simulink model "ModeloUnaOruga"  (R2023b)
settings: Solver=VariableStepAuto  StartTime=0.0  StopTime=10  RelTol=1e-3
model workspace: external: MATLAB File C:\Users\marco\MATLAB\Projects\SimulacionOrugas\Ensamblaje_Sim_v8_DataFile.m (data not in the file)
undefined symbols (not defined in the file or in its folder): smiData, X, Y, Z
libraries: sm_lib x1001, nesl_utility x3, simulink x1
(part 5 of 16)

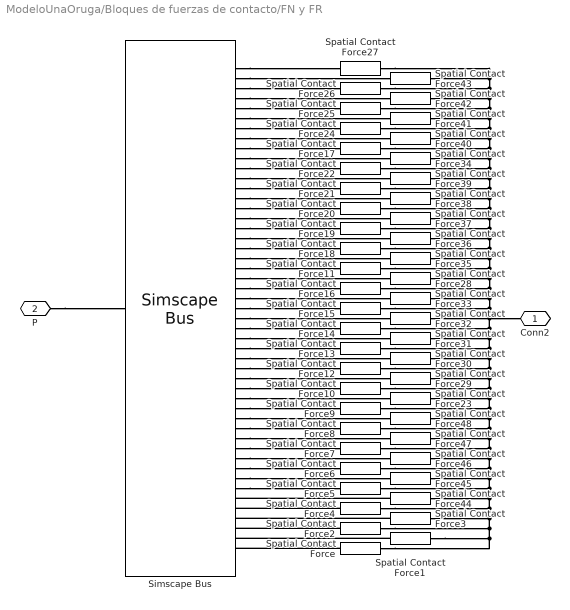
== system ModeloUnaOruga/Bloques de fuerzas de contacto/FN y FR ==
  Simscape Bus : SimscapeBus  HierarchyStrings=Connection49;Connection48;Connection47;Connection46;Connection45;Connection44;Connection43;Connection42;Connection41;Connection40;Connection39;Connection38;Connection37;Connection36;Connection35;Connection34;Connection33;Connection32;Connection31;Connection30;Connection29;Connection28;Connection27;Connection26;Connection25;Connection24;Connection23;Connection22;Connection21;Connection20;Connection19;Connection18;Connection17;Connection16;Connection15;Connection14;Connection13;Connection12;Connection11;Connection10;Connection9;Connection8;Connection7;Connection6;Connection5;Connection4;Connection3;Connection2;Connection1
  Spatial Contact Force{,1..48} (49 alike) : sm_lib/Forces and Torques/Spatial Contact Force  SenseContactBaseRotation=off  SenseContactBaseTranslation=off  CoefficientOfDynamicFriction=0.3  CoefficientOfStaticFriction=0.5  NormalDamping=1e3  NormalDampingUnits=N/(m/s)  SenseContactSignal=off  NormalStiffness=1e6  NormalStiffnessUnits=N/m  FrictionalCriticalVelocity=1e-3  FrictionalCriticalVelocityUnits=m/s  ZeroCrossDetectContactStartAndEnd=off  SenseContactFollowerRotation=off  SenseContactFollowerTranslation=off  FrictionType=SmoothStickSlip  SenseFrictionalForceMagnitude=off  SenseNormalForceMagnitude=off  NormalForceType=SmoothSpringDamper  SenseNormalVelocity=off  SensePenetrationDepth=off  SenseSeparationDistance=off  SenseTangentialVelocity=off  NormalTransitionRegionWidth=1e-4  NormalTransitionRegionWidthUnits=m
  Conn2 : PMIOPort  Side=Right
  P : PMIOPort  Port=2  Side=Left
  connections:
  Spatial Contact Force/RConn1 -- Spatial Contact Force1/RConn1 -- Spatial Contact Force2/RConn1 -- Spatial Contact Force3/RConn1 -- Spatial Contact Force4/RConn1 -- Spatial Contact Force44/RConn1 -- Spatial Contact Force5/RConn1 -- Spatial Contact Force45/RConn1 -- Spatial Contact Force6/RConn1 -- Spatial Contact Force46/RConn1 -- Spatial Contact Force7/RConn1 -- Spatial Contact Force47/RConn1 -- Spatial Contact Force8/RConn1 -- Spatial Contact Force48/RConn1 -- Spatial Contact Force9/RConn1 -- Spatial Contact Force23/RConn1 -- Spatial Contact Force10/RConn1 -- Spatial Contact Force29/RConn1 -- Spatial Contact Force12/RConn1 -- Spatial Contact Force30/RConn1 -- Spatial Contact Force13/RConn1 -- Spatial Contact Force31/RConn1 -- Spatial Contact Force14/RConn1 -- Spatial Contact Force18/RConn1 -- Spatial Contact Force43/RConn1 -- Spatial Contact Force27/RConn1 -- Spatial Contact Force26/RConn1 -- Spatial Contact Force42/RConn1 -- Spatial Contact Force25/RConn1 -- Spatial Contact Force41/RConn1 -- Spatial Contact Force24/RConn1 -- Spatial Contact Force40/RConn1 -- Spatial Contact Force17/RConn1 -- Spatial Contact Force34/RConn1 -- Spatial Contact Force22/RConn1 -- Spatial Contact Force39/RConn1 -- Spatial Contact Force21/RConn1 -- Spatial Contact Force38/RConn1 -- Spatial Contact Force20/RConn1 -- Spatial Contact Force37/RConn1 -- Spatial Contact Force19/RConn1 -- Spatial Contact Force36/RConn1 -- Spatial Contact Force35/RConn1 -- Spatial Contact Force11/RConn1 -- Spatial Contact Force28/RConn1 -- Spatial Contact Force16/RConn1 -- Spatial Contact Force33/RConn1 -- Spatial Contact Force15/RConn1 -- Spatial Contact Force32/RConn1 -- Conn2/RConn1
  Spatial Contact Force/LConn1 -- Simscape Bus/LConn49
  Spatial Contact Force1/LConn1 -- Simscape Bus/LConn48
  Spatial Contact Force2/LConn1 -- Simscape Bus/LConn47
  Spatial Contact Force3/LConn1 -- Simscape Bus/LConn46
  Spatial Contact Force4/LConn1 -- Simscape Bus/LConn45
  Spatial Contact Force44/LConn1 -- Simscape Bus/LConn44
  Simscape Bus/LConn43 -- Spatial Contact Force5/LConn1
  Simscape Bus/LConn42 -- Spatial Contact Force45/LConn1
  Simscape Bus/LConn41 -- Spatial Contact Force6/LConn1
  Simscape Bus/LConn40 -- Spatial Contact Force46/LConn1
  Simscape Bus/LConn39 -- Spatial Contact Force7/LConn1
  Simscape Bus/LConn38 -- Spatial Contact Force47/LConn1
  Simscape Bus/LConn37 -- Spatial Contact Force8/LConn1
  Simscape Bus/LConn36 -- Spatial Contact Force48/LConn1
  Simscape Bus/LConn35 -- Spatial Contact Force9/LConn1
  Simscape Bus/LConn34 -- Spatial Contact Force23/LConn1
  Simscape Bus/LConn33 -- Spatial Contact Force10/LConn1
  Simscape Bus/LConn32 -- Spatial Contact Force29/LConn1
  Simscape Bus/LConn31 -- Spatial Contact Force12/LConn1
  Simscape Bus/LConn30 -- Spatial Contact Force30/LConn1
  Simscape Bus/LConn29 -- Spatial Contact Force13/LConn1
  Simscape Bus/LConn28 -- Spatial Contact Force31/LConn1
  Simscape Bus/LConn27 -- Spatial Contact Force14/LConn1
  Simscape Bus/LConn26 -- Spatial Contact Force32/LConn1
  Simscape Bus/LConn25 -- Spatial Contact Force15/LConn1
  Simscape Bus/LConn24 -- Spatial Contact Force33/LConn1
  Simscape Bus/LConn23 -- Spatial Contact Force16/LConn1
  Simscape Bus/LConn22 -- Spatial Contact Force28/LConn1
  Simscape Bus/LConn21 -- Spatial Contact Force11/LConn1
  Simscape Bus/LConn20 -- Spatial Contact Force35/LConn1
  Simscape Bus/LConn19 -- Spatial Contact Force18/LConn1
  Simscape Bus/LConn18 -- Spatial Contact Force36/LConn1
  Simscape Bus/LConn17 -- Spatial Contact Force19/LConn1
  Simscape Bus/LConn16 -- Spatial Contact Force37/LConn1
  Simscape Bus/LConn15 -- Spatial Contact Force20/LConn1
  Simscape Bus/LConn14 -- Spatial Contact Force38/LConn1
  Simscape Bus/LConn13 -- Spatial Contact Force21/LConn1
  Simscape Bus/LConn12 -- Spatial Contact Force39/LConn1
  Simscape Bus/LConn11 -- Spatial Contact Force22/LConn1
  Simscape Bus/LConn10 -- Spatial Contact Force34/LConn1
  Simscape Bus/LConn9 -- Spatial Contact Force17/LConn1
  Simscape Bus/LConn8 -- Spatial Contact Force40/LConn1
  Simscape Bus/LConn7 -- Spatial Contact Force24/LConn1
  Simscape Bus/LConn6 -- Spatial Contact Force41/LConn1
  Simscape Bus/LConn5 -- Spatial Contact Force25/LConn1
  Simscape Bus/LConn4 -- Spatial Contact Force42/LConn1
  Simscape Bus/LConn3 -- Spatial Contact Force26/LConn1
  Simscape Bus/LConn2 -- Spatial Contact Force43/LConn1
  Simscape Bus/LConn1 -- Spatial Contact Force27/LConn1
  P/RConn1 -- Simscape Bus/RConn1

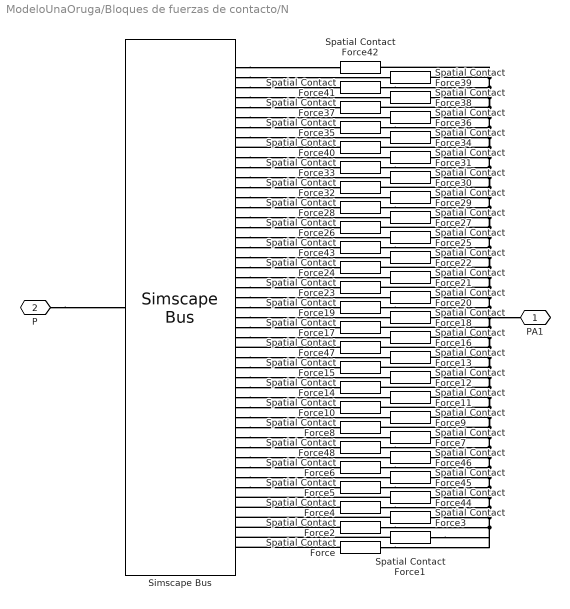
== system ModeloUnaOruga/Bloques de fuerzas de contacto/N ==
  Simscape Bus : SimscapeBus  HierarchyStrings=Connection49;Connection48;Connection47;Connection46;Connection45;Connection44;Connection43;Connection42;Connection41;Connection40;Connection39;Connection38;Connection37;Connection36;Connection35;Connection34;Connection33;Connection32;Connection31;Connection30;Connection29;Connection28;Connection27;Connection26;Connection25;Connection24;Connection23;Connection22;Connection21;Connection20;Connection19;Connection18;Connection17;Connection16;Connection15;Connection14;Connection13;Connection12;Connection11;Connection10;Connection9;Connection8;Connection7;Connection6;Connection5;Connection4;Connection3;Connection2;Connection1
  Spatial Contact Force{,1..48} (49 alike) : sm_lib/Forces and Torques/Spatial Contact Force  SenseContactBaseRotation=off  SenseContactBaseTranslation=off  CoefficientOfDynamicFriction=0.3  CoefficientOfStaticFriction=0.5  NormalDamping=1e3  NormalDampingUnits=N/(m/s)  SenseContactSignal=off  NormalStiffness=1e6  NormalStiffnessUnits=N/m  FrictionalCriticalVelocity=1e-3  FrictionalCriticalVelocityUnits=m/s  ZeroCrossDetectContactStartAndEnd=off  SenseContactFollowerRotation=off  SenseContactFollowerTranslation=off  FrictionType=None  SenseFrictionalForceMagnitude=off  SenseNormalForceMagnitude=off  NormalForceType=SmoothSpringDamper  SenseNormalVelocity=off  SensePenetrationDepth=off  SenseSeparationDistance=off  SenseTangentialVelocity=off  NormalTransitionRegionWidth=1e-4  NormalTransitionRegionWidthUnits=m
  PA1 : PMIOPort  Side=Right
  P : PMIOPort  Port=2  Side=Left
  connections:
  Spatial Contact Force41/RConn1 -- Spatial Contact Force38/RConn1 -- Spatial Contact Force35/RConn1 -- Spatial Contact Force28/RConn1 -- Spatial Contact Force46/RConn1 -- Spatial Contact Force6/RConn1 -- Spatial Contact Force45/RConn1 -- Spatial Contact Force5/RConn1 -- Spatial Contact Force44/RConn1 -- Spatial Contact Force1/RConn1 -- Spatial Contact Force/RConn1 -- Spatial Contact Force2/RConn1 -- Spatial Contact Force3/RConn1 -- Spatial Contact Force4/RConn1 -- Spatial Contact Force48/RConn1 -- Spatial Contact Force7/RConn1 -- Spatial Contact Force8/RConn1 -- Spatial Contact Force9/RConn1 -- Spatial Contact Force10/RConn1 -- Spatial Contact Force11/RConn1 -- Spatial Contact Force14/RConn1 -- Spatial Contact Force12/RConn1 -- Spatial Contact Force15/RConn1 -- Spatial Contact Force13/RConn1 -- Spatial Contact Force47/RConn1 -- Spatial Contact Force16/RConn1 -- Spatial Contact Force17/RConn1 -- Spatial Contact Force18/RConn1 -- PA1/RConn1 -- Spatial Contact Force19/RConn1 -- Spatial Contact Force20/RConn1 -- Spatial Contact Force23/RConn1 -- Spatial Contact Force21/RConn1 -- Spatial Contact Force24/RConn1 -- Spatial Contact Force22/RConn1 -- Spatial Contact Force43/RConn1 -- Spatial Contact Force25/RConn1 -- Spatial Contact Force26/RConn1 -- Spatial Contact Force27/RConn1 -- Spatial Contact Force29/RConn1 -- Spatial Contact Force32/RConn1 -- Spatial Contact Force30/RConn1 -- Spatial Contact Force33/RConn1 -- Spatial Contact Force31/RConn1 -- Spatial Contact Force40/RConn1 -- Spatial Contact Force34/RConn1 -- Spatial Contact Force36/RConn1 -- Spatial Contact Force37/RConn1 -- Spatial Contact Force42/RConn1 -- Spatial Contact Force39/RConn1
  Spatial Contact Force/LConn1 -- Simscape Bus/LConn49
  Spatial Contact Force1/LConn1 -- Simscape Bus/LConn48
  Spatial Contact Force2/LConn1 -- Simscape Bus/LConn47
  Spatial Contact Force3/LConn1 -- Simscape Bus/LConn46
  Spatial Contact Force4/LConn1 -- Simscape Bus/LConn45
  Spatial Contact Force44/LConn1 -- Simscape Bus/LConn44
  Simscape Bus/LConn43 -- Spatial Contact Force5/LConn1
  Simscape Bus/LConn42 -- Spatial Contact Force45/LConn1
  Simscape Bus/LConn41 -- Spatial Contact Force6/LConn1
  Simscape Bus/LConn40 -- Spatial Contact Force46/LConn1
  P/RConn1 -- Simscape Bus/RConn1
  Simscape Bus/LConn36 -- Spatial Contact Force9/LConn1
  Simscape Bus/LConn37 -- Spatial Contact Force8/LConn1
  Simscape Bus/LConn32 -- Spatial Contact Force12/LConn1
  Simscape Bus/LConn30 -- Spatial Contact Force13/LConn1
  Simscape Bus/LConn38 -- Spatial Contact Force7/LConn1
  Simscape Bus/LConn31 -- Spatial Contact Force15/LConn1
  Simscape Bus/LConn35 -- Spatial Contact Force10/LConn1
  Simscape Bus/LConn33 -- Spatial Contact Force14/LConn1
  Simscape Bus/LConn34 -- Spatial Contact Force11/LConn1
  Simscape Bus/LConn26 -- Spatial Contact Force18/LConn1
  Simscape Bus/LConn27 -- Spatial Contact Force17/LConn1
  Simscape Bus/LConn22 -- Spatial Contact Force21/LConn1
  Simscape Bus/LConn20 -- Spatial Contact Force22/LConn1
  Simscape Bus/LConn28 -- Spatial Contact Force16/LConn1
  Simscape Bus/LConn21 -- Spatial Contact Force24/LConn1
  Simscape Bus/LConn25 -- Spatial Contact Force19/LConn1
  Simscape Bus/LConn23 -- Spatial Contact Force23/LConn1
  Simscape Bus/LConn24 -- Spatial Contact Force20/LConn1
  Simscape Bus/LConn16 -- Spatial Contact Force27/LConn1
  Simscape Bus/LConn17 -- Spatial Contact Force26/LConn1
  Simscape Bus/LConn12 -- Spatial Contact Force30/LConn1
  Simscape Bus/LConn10 -- Spatial Contact Force31/LConn1
  Simscape Bus/LConn18 -- Spatial Contact Force25/LConn1
  Simscape Bus/LConn11 -- Spatial Contact Force33/LConn1
  Simscape Bus/LConn15 -- Spatial Contact Force28/LConn1
  Simscape Bus/LConn13 -- Spatial Contact Force32/LConn1
  Simscape Bus/LConn14 -- Spatial Contact Force29/LConn1
  Simscape Bus/LConn6 -- Spatial Contact Force36/LConn1
  Simscape Bus/LConn7 -- Spatial Contact Force35/LConn1
  Simscape Bus/LConn2 -- Spatial Contact Force39/LConn1
  Simscape Bus/LConn8 -- Spatial Contact Force34/LConn1
  Simscape Bus/LConn1 -- Spatial Contact Force42/LConn1
  Simscape Bus/LConn5 -- Spatial Contact Force37/LConn1
  Simscape Bus/LConn3 -- Spatial Contact Force41/LConn1
  Simscape Bus/LConn4 -- Spatial Contact Force38/LConn1
  Spatial Contact Force40/LConn1 -- Simscape Bus/LConn9
  Simscape Bus/LConn19 -- Spatial Contact Force43/LConn1
  Spatial Contact Force47/LConn1 -- Simscape Bus/LConn29
  Simscape Bus/LConn39 -- Spatial Contact Force48/LConn1

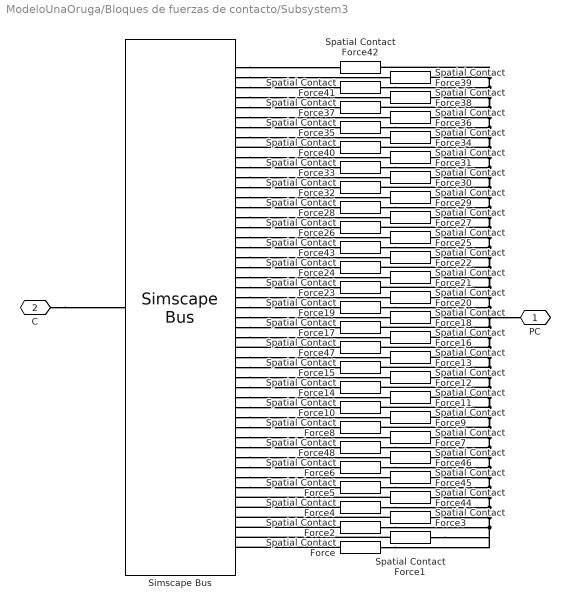
== system ModeloUnaOruga/Bloques de fuerzas de contacto/Subsystem3 ==
  Simscape Bus : SimscapeBus  HierarchyStrings=Connection49;Connection48;Connection47;Connection46;Connection45;Connection44;Connection43;Connection42;Connection41;Connection40;Connection39;Connection38;Connection37;Connection36;Connection35;Connection34;Connection33;Connection32;Connection31;Connection30;Connection29;Connection28;Connection27;Connection26;Connection25;Connection24;Connection23;Connection22;Connection21;Connection20;Connection19;Connection18;Connection17;Connection16;Connection15;Connection14;Connection13;Connection12;Connection11;Connection10;Connection9;Connection8;Connection7;Connection6;Connection5;Connection4;Connection3;Connection2;Connection1
  Spatial Contact Force{,1..48} (49 alike) : sm_lib/Forces and Torques/Spatial Contact Force  SenseContactBaseRotation=off  SenseContactBaseTranslation=off  CoefficientOfDynamicFriction=0.3  CoefficientOfStaticFriction=0.5  NormalDamping=1e3  NormalDampingUnits=N/(m/s)  SenseContactSignal=off  NormalStiffness=1e6  NormalStiffnessUnits=N/m  FrictionalCriticalVelocity=1e-3  FrictionalCriticalVelocityUnits=m/s  ZeroCrossDetectContactStartAndEnd=off  SenseContactFollowerRotation=off  SenseContactFollowerTranslation=off  FrictionType=None  SenseFrictionalForceMagnitude=off  SenseNormalForceMagnitude=off  NormalForceType=SmoothSpringDamper  SenseNormalVelocity=off  SensePenetrationDepth=off  SenseSeparationDistance=off  SenseTangentialVelocity=off  NormalTransitionRegionWidth=1e-4  NormalTransitionRegionWidthUnits=m
  PC : PMIOPort  Side=Right
  C : PMIOPort  Port=2  Side=Left
  connections:
  Spatial Contact Force41/RConn1 -- Spatial Contact Force42/RConn1 -- Spatial Contact Force39/RConn1 -- Spatial Contact Force38/RConn1 -- Spatial Contact Force35/RConn1 -- Spatial Contact Force40/RConn1 -- Spatial Contact Force32/RConn1 -- Spatial Contact Force28/RConn1 -- Spatial Contact Force26/RConn1 -- Spatial Contact Force24/RConn1 -- Spatial Contact Force23/RConn1 -- Spatial Contact Force17/RConn1 -- Spatial Contact Force16/RConn1 -- Spatial Contact Force47/RConn1 -- Spatial Contact Force13/RConn1 -- Spatial Contact Force15/RConn1 -- Spatial Contact Force14/RConn1 -- Spatial Contact Force11/RConn1 -- Spatial Contact Force10/RConn1 -- Spatial Contact Force9/RConn1 -- Spatial Contact Force8/RConn1 -- Spatial Contact Force46/RConn1 -- Spatial Contact Force6/RConn1 -- Spatial Contact Force45/RConn1 -- Spatial Contact Force5/RConn1 -- Spatial Contact Force44/RConn1 -- Spatial Contact Force1/RConn1 -- Spatial Contact Force/RConn1 -- Spatial Contact Force2/RConn1 -- Spatial Contact Force3/RConn1 -- Spatial Contact Force4/RConn1 -- Spatial Contact Force48/RConn1 -- Spatial Contact Force7/RConn1 -- Spatial Contact Force12/RConn1 -- Spatial Contact Force18/RConn1 -- PC/RConn1 -- Spatial Contact Force19/RConn1 -- Spatial Contact Force20/RConn1 -- Spatial Contact Force21/RConn1 -- Spatial Contact Force22/RConn1 -- Spatial Contact Force43/RConn1 -- Spatial Contact Force25/RConn1 -- Spatial Contact Force27/RConn1 -- Spatial Contact Force29/RConn1 -- Spatial Contact Force30/RConn1 -- Spatial Contact Force33/RConn1 -- Spatial Contact Force31/RConn1 -- Spatial Contact Force34/RConn1 -- Spatial Contact Force36/RConn1 -- Spatial Contact Force37/RConn1
  Spatial Contact Force/LConn1 -- Simscape Bus/LConn49
  Spatial Contact Force1/LConn1 -- Simscape Bus/LConn48
  Spatial Contact Force2/LConn1 -- Simscape Bus/LConn47
  Spatial Contact Force3/LConn1 -- Simscape Bus/LConn46
  Spatial Contact Force4/LConn1 -- Simscape Bus/LConn45
  Spatial Contact Force44/LConn1 -- Simscape Bus/LConn44
  Simscape Bus/LConn43 -- Spatial Contact Force5/LConn1
  Simscape Bus/LConn42 -- Spatial Contact Force45/LConn1
  Simscape Bus/LConn41 -- Spatial Contact Force6/LConn1
  Simscape Bus/LConn40 -- Spatial Contact Force46/LConn1
  C/RConn1 -- Simscape Bus/RConn1
  Simscape Bus/LConn36 -- Spatial Contact Force9/LConn1
  Simscape Bus/LConn37 -- Spatial Contact Force8/LConn1
  Simscape Bus/LConn32 -- Spatial Contact Force12/LConn1
  Simscape Bus/LConn30 -- Spatial Contact Force13/LConn1
  Simscape Bus/LConn38 -- Spatial Contact Force7/LConn1
  Simscape Bus/LConn31 -- Spatial Contact Force15/LConn1
  Simscape Bus/LConn35 -- Spatial Contact Force10/LConn1
  Simscape Bus/LConn33 -- Spatial Contact Force14/LConn1
  Simscape Bus/LConn34 -- Spatial Contact Force11/LConn1
  Simscape Bus/LConn26 -- Spatial Contact Force18/LConn1
  Simscape Bus/LConn27 -- Spatial Contact Force17/LConn1
  Simscape Bus/LConn22 -- Spatial Contact Force21/LConn1
  Simscape Bus/LConn20 -- Spatial Contact Force22/LConn1
  Simscape Bus/LConn28 -- Spatial Contact Force16/LConn1
  Simscape Bus/LConn21 -- Spatial Contact Force24/LConn1
  Simscape Bus/LConn25 -- Spatial Contact Force19/LConn1
  Simscape Bus/LConn23 -- Spatial Contact Force23/LConn1
  Simscape Bus/LConn24 -- Spatial Contact Force20/LConn1
  Simscape Bus/LConn16 -- Spatial Contact Force27/LConn1
  Simscape Bus/LConn17 -- Spatial Contact Force26/LConn1
  Simscape Bus/LConn12 -- Spatial Contact Force30/LConn1
  Simscape Bus/LConn10 -- Spatial Contact Force31/LConn1
  Simscape Bus/LConn18 -- Spatial Contact Force25/LConn1
  Simscape Bus/LConn11 -- Spatial Contact Force33/LConn1
  Simscape Bus/LConn15 -- Spatial Contact Force28/LConn1
  Simscape Bus/LConn13 -- Spatial Contact Force32/LConn1
  Simscape Bus/LConn14 -- Spatial Contact Force29/LConn1
  Simscape Bus/LConn6 -- Spatial Contact Force36/LConn1
  Simscape Bus/LConn7 -- Spatial Contact Force35/LConn1
  Simscape Bus/LConn2 -- Spatial Contact Force39/LConn1
  Simscape Bus/LConn8 -- Spatial Contact Force34/LConn1
  Simscape Bus/LConn1 -- Spatial Contact Force42/LConn1
  Simscape Bus/LConn5 -- Spatial Contact Force37/LConn1
  Simscape Bus/LConn3 -- Spatial Contact Force41/LConn1
  Simscape Bus/LConn4 -- Spatial Contact Force38/LConn1
  Spatial Contact Force40/LConn1 -- Simscape Bus/LConn9
  Simscape Bus/LConn19 -- Spatial Contact Force43/LConn1
  Spatial Contact Force47/LConn1 -- Simscape Bus/LConn29
  Simscape Bus/LConn39 -- Spatial Contact Force48/LConn1

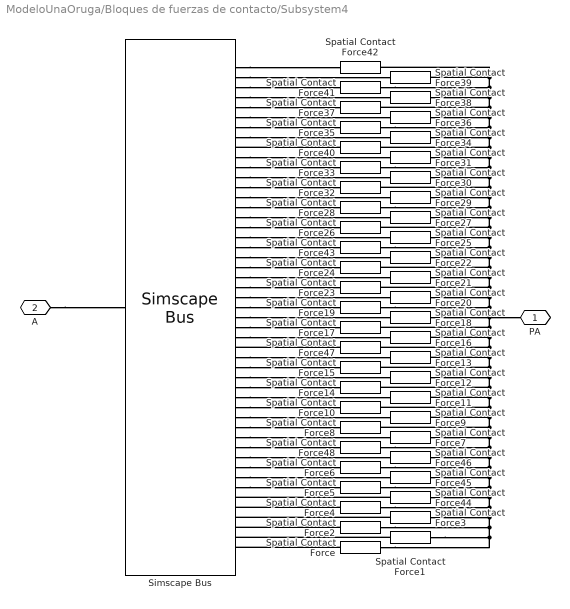
== system ModeloUnaOruga/Bloques de fuerzas de contacto/Subsystem4 ==
  Simscape Bus : SimscapeBus  HierarchyStrings=Connection49;Connection48;Connection47;Connection46;Connection45;Connection44;Connection43;Connection42;Connection41;Connection40;Connection39;Connection38;Connection37;Connection36;Connection35;Connection34;Connection33;Connection32;Connection31;Connection30;Connection29;Connection28;Connection27;Connection26;Connection25;Connection24;Connection23;Connection22;Connection21;Connection20;Connection19;Connection18;Connection17;Connection16;Connection15;Connection14;Connection13;Connection12;Connection11;Connection10;Connection9;Connection8;Connection7;Connection6;Connection5;Connection4;Connection3;Connection2;Connection1
  Spatial Contact Force{,1..48} (49 alike) : sm_lib/Forces and Torques/Spatial Contact Force  SenseContactBaseRotation=off  SenseContactBaseTranslation=off  CoefficientOfDynamicFriction=0.3  CoefficientOfStaticFriction=0.5  NormalDamping=1e3  NormalDampingUnits=N/(m/s)  SenseContactSignal=off  NormalStiffness=1e6  NormalStiffnessUnits=N/m  FrictionalCriticalVelocity=1e-3  FrictionalCriticalVelocityUnits=m/s  ZeroCrossDetectContactStartAndEnd=off  SenseContactFollowerRotation=off  SenseContactFollowerTranslation=off  FrictionType=None  SenseFrictionalForceMagnitude=off  SenseNormalForceMagnitude=off  NormalForceType=SmoothSpringDamper  SenseNormalVelocity=off  SensePenetrationDepth=off  SenseSeparationDistance=off  SenseTangentialVelocity=off  NormalTransitionRegionWidth=1e-4  NormalTransitionRegionWidthUnits=m
  PA : PMIOPort  Side=Right
  A : PMIOPort  Port=2  Side=Left
  connections:
  Spatial Contact Force46/RConn1 -- Spatial Contact Force6/RConn1 -- Spatial Contact Force45/RConn1 -- Spatial Contact Force5/RConn1 -- Spatial Contact Force44/RConn1 -- Spatial Contact Force1/RConn1 -- Spatial Contact Force/RConn1 -- Spatial Contact Force2/RConn1 -- Spatial Contact Force3/RConn1 -- Spatial Contact Force4/RConn1 -- Spatial Contact Force48/RConn1 -- Spatial Contact Force7/RConn1 -- Spatial Contact Force8/RConn1 -- Spatial Contact Force9/RConn1 -- Spatial Contact Force10/RConn1 -- Spatial Contact Force11/RConn1 -- Spatial Contact Force14/RConn1 -- Spatial Contact Force12/RConn1 -- Spatial Contact Force15/RConn1 -- Spatial Contact Force13/RConn1 -- Spatial Contact Force47/RConn1 -- Spatial Contact Force16/RConn1 -- Spatial Contact Force17/RConn1 -- Spatial Contact Force19/RConn1 -- Spatial Contact Force20/RConn1 -- Spatial Contact Force23/RConn1 -- Spatial Contact Force24/RConn1 -- Spatial Contact Force22/RConn1 -- Spatial Contact Force43/RConn1 -- Spatial Contact Force26/RConn1 -- Spatial Contact Force32/RConn1 -- Spatial Contact Force30/RConn1 -- Spatial Contact Force33/RConn1 -- Spatial Contact Force31/RConn1 -- Spatial Contact Force40/RConn1 -- Spatial Contact Force35/RConn1 -- Spatial Contact Force37/RConn1 -- Spatial Contact Force41/RConn1 -- Spatial Contact Force42/RConn1 -- Spatial Contact Force39/RConn1 -- Spatial Contact Force38/RConn1 -- Spatial Contact Force36/RConn1 -- Spatial Contact Force34/RConn1 -- Spatial Contact Force29/RConn1 -- Spatial Contact Force28/RConn1 -- Spatial Contact Force27/RConn1 -- Spatial Contact Force25/RConn1 -- Spatial Contact Force21/RConn1 -- Spatial Contact Force18/RConn1 -- PA/RConn1
  Spatial Contact Force/LConn1 -- Simscape Bus/LConn49
  Spatial Contact Force1/LConn1 -- Simscape Bus/LConn48
  Spatial Contact Force2/LConn1 -- Simscape Bus/LConn47
  Spatial Contact Force3/LConn1 -- Simscape Bus/LConn46
  Spatial Contact Force4/LConn1 -- Simscape Bus/LConn45
  Spatial Contact Force44/LConn1 -- Simscape Bus/LConn44
  Simscape Bus/LConn43 -- Spatial Contact Force5/LConn1
  Simscape Bus/LConn42 -- Spatial Contact Force45/LConn1
  Simscape Bus/LConn41 -- Spatial Contact Force6/LConn1
  Simscape Bus/LConn40 -- Spatial Contact Force46/LConn1
  A/RConn1 -- Simscape Bus/RConn1
  Simscape Bus/LConn36 -- Spatial Contact Force9/LConn1
  Simscape Bus/LConn37 -- Spatial Contact Force8/LConn1
  Simscape Bus/LConn32 -- Spatial Contact Force12/LConn1
  Simscape Bus/LConn30 -- Spatial Contact Force13/LConn1
  Simscape Bus/LConn38 -- Spatial Contact Force7/LConn1
  Simscape Bus/LConn31 -- Spatial Contact Force15/LConn1
  Simscape Bus/LConn35 -- Spatial Contact Force10/LConn1
  Simscape Bus/LConn33 -- Spatial Contact Force14/LConn1
  Simscape Bus/LConn34 -- Spatial Contact Force11/LConn1
  Simscape Bus/LConn26 -- Spatial Contact Force18/LConn1
  Simscape Bus/LConn27 -- Spatial Contact Force17/LConn1
  Simscape Bus/LConn22 -- Spatial Contact Force21/LConn1
  Simscape Bus/LConn20 -- Spatial Contact Force22/LConn1
  Simscape Bus/LConn28 -- Spatial Contact Force16/LConn1
  Simscape Bus/LConn21 -- Spatial Contact Force24/LConn1
  Simscape Bus/LConn25 -- Spatial Contact Force19/LConn1
  Simscape Bus/LConn23 -- Spatial Contact Force23/LConn1
  Simscape Bus/LConn24 -- Spatial Contact Force20/LConn1
  Simscape Bus/LConn16 -- Spatial Contact Force27/LConn1
  Simscape Bus/LConn17 -- Spatial Contact Force26/LConn1
  Simscape Bus/LConn12 -- Spatial Contact Force30/LConn1
  Simscape Bus/LConn10 -- Spatial Contact Force31/LConn1
  Simscape Bus/LConn18 -- Spatial Contact Force25/LConn1
  Simscape Bus/LConn11 -- Spatial Contact Force33/LConn1
  Simscape Bus/LConn15 -- Spatial Contact Force28/LConn1
  Simscape Bus/LConn13 -- Spatial Contact Force32/LConn1
  Simscape Bus/LConn14 -- Spatial Contact Force29/LConn1
  Simscape Bus/LConn6 -- Spatial Contact Force36/LConn1
  Simscape Bus/LConn7 -- Spatial Contact Force35/LConn1
  Simscape Bus/LConn2 -- Spatial Contact Force39/LConn1
  Simscape Bus/LConn8 -- Spatial Contact Force34/LConn1
  Simscape Bus/LConn1 -- Spatial Contact Force42/LConn1
  Simscape Bus/LConn5 -- Spatial Contact Force37/LConn1
  Simscape Bus/LConn3 -- Spatial Contact Force41/LConn1
  Simscape Bus/LConn4 -- Spatial Contact Force38/LConn1
  Spatial Contact Force40/LConn1 -- Simscape Bus/LConn9
  Simscape Bus/LConn19 -- Spatial Contact Force43/LConn1
  Spatial Contact Force47/LConn1 -- Simscape Bus/LConn29
  Simscape Bus/LConn39 -- Spatial Contact Force48/LConn1

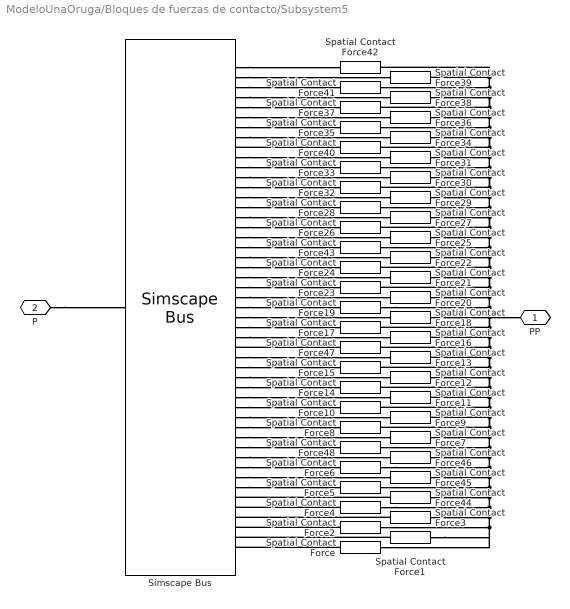
== system ModeloUnaOruga/Bloques de fuerzas de contacto/Subsystem5 ==
  Simscape Bus : SimscapeBus  HierarchyStrings=Connection49;Connection48;Connection47;Connection46;Connection45;Connection44;Connection43;Connection42;Connection41;Connection40;Connection39;Connection38;Connection37;Connection36;Connection35;Connection34;Connection33;Connection32;Connection31;Connection30;Connection29;Connection28;Connection27;Connection26;Connection25;Connection24;Connection23;Connection22;Connection21;Connection20;Connection19;Connection18;Connection17;Connection16;Connection15;Connection14;Connection13;Connection12;Connection11;Connection10;Connection9;Connection8;Connection7;Connection6;Connection5;Connection4;Connection3;Connection2;Connection1
  Spatial Contact Force{,1..48} (49 alike) : sm_lib/Forces and Torques/Spatial Contact Force  SenseContactBaseRotation=off  SenseContactBaseTranslation=off  CoefficientOfDynamicFriction=0.3  CoefficientOfStaticFriction=0.5  NormalDamping=1e3  NormalDampingUnits=N/(m/s)  SenseContactSignal=off  NormalStiffness=1e6  NormalStiffnessUnits=N/m  FrictionalCriticalVelocity=1e-3  FrictionalCriticalVelocityUnits=m/s  ZeroCrossDetectContactStartAndEnd=off  SenseContactFollowerRotation=off  SenseContactFollowerTranslation=off  FrictionType=None  SenseFrictionalForceMagnitude=off  SenseNormalForceMagnitude=off  NormalForceType=SmoothSpringDamper  SenseNormalVelocity=off  SensePenetrationDepth=off  SenseSeparationDistance=off  SenseTangentialVelocity=off  NormalTransitionRegionWidth=1e-4  NormalTransitionRegionWidthUnits=m
  PP : PMIOPort  Side=Right
  P : PMIOPort  Port=2  Side=Left
  connections:
  Spatial Contact Force41/RConn1 -- Spatial Contact Force42/RConn1 -- Spatial Contact Force39/RConn1 -- Spatial Contact Force38/RConn1 -- Spatial Contact Force35/RConn1 -- Spatial Contact Force40/RConn1 -- Spatial Contact Force32/RConn1 -- Spatial Contact Force28/RConn1 -- Spatial Contact Force26/RConn1 -- Spatial Contact Force24/RConn1 -- Spatial Contact Force23/RConn1 -- Spatial Contact Force17/RConn1 -- Spatial Contact Force16/RConn1 -- Spatial Contact Force47/RConn1 -- Spatial Contact Force13/RConn1 -- Spatial Contact Force15/RConn1 -- Spatial Contact Force14/RConn1 -- Spatial Contact Force11/RConn1 -- Spatial Contact Force10/RConn1 -- Spatial Contact Force9/RConn1 -- Spatial Contact Force8/RConn1 -- Spatial Contact Force46/RConn1 -- Spatial Contact Force6/RConn1 -- Spatial Contact Force45/RConn1 -- Spatial Contact Force5/RConn1 -- Spatial Contact Force44/RConn1 -- Spatial Contact Force1/RConn1 -- Spatial Contact Force/RConn1 -- Spatial Contact Force2/RConn1 -- Spatial Contact Force3/RConn1 -- Spatial Contact Force4/RConn1 -- Spatial Contact Force48/RConn1 -- Spatial Contact Force7/RConn1 -- Spatial Contact Force12/RConn1 -- Spatial Contact Force18/RConn1 -- PP/RConn1 -- Spatial Contact Force19/RConn1 -- Spatial Contact Force20/RConn1 -- Spatial Contact Force21/RConn1 -- Spatial Contact Force22/RConn1 -- Spatial Contact Force43/RConn1 -- Spatial Contact Force25/RConn1 -- Spatial Contact Force27/RConn1 -- Spatial Contact Force29/RConn1 -- Spatial Contact Force30/RConn1 -- Spatial Contact Force33/RConn1 -- Spatial Contact Force31/RConn1 -- Spatial Contact Force34/RConn1 -- Spatial Contact Force36/RConn1 -- Spatial Contact Force37/RConn1
  Spatial Contact Force/LConn1 -- Simscape Bus/LConn49
  Spatial Contact Force1/LConn1 -- Simscape Bus/LConn48
  Spatial Contact Force2/LConn1 -- Simscape Bus/LConn47
  Spatial Contact Force3/LConn1 -- Simscape Bus/LConn46
  Spatial Contact Force4/LConn1 -- Simscape Bus/LConn45
  Spatial Contact Force44/LConn1 -- Simscape Bus/LConn44
  Simscape Bus/LConn43 -- Spatial Contact Force5/LConn1
  Simscape Bus/LConn42 -- Spatial Contact Force45/LConn1
  Simscape Bus/LConn41 -- Spatial Contact Force6/LConn1
  Simscape Bus/LConn40 -- Spatial Contact Force46/LConn1
  P/RConn1 -- Simscape Bus/RConn1
  Simscape Bus/LConn36 -- Spatial Contact Force9/LConn1
  Simscape Bus/LConn37 -- Spatial Contact Force8/LConn1
  Simscape Bus/LConn32 -- Spatial Contact Force12/LConn1
  Simscape Bus/LConn30 -- Spatial Contact Force13/LConn1
  Simscape Bus/LConn38 -- Spatial Contact Force7/LConn1
  Simscape Bus/LConn31 -- Spatial Contact Force15/LConn1
  Simscape Bus/LConn35 -- Spatial Contact Force10/LConn1
  Simscape Bus/LConn33 -- Spatial Contact Force14/LConn1
  Simscape Bus/LConn34 -- Spatial Contact Force11/LConn1
  Simscape Bus/LConn26 -- Spatial Contact Force18/LConn1
  Simscape Bus/LConn27 -- Spatial Contact Force17/LConn1
  Simscape Bus/LConn22 -- Spatial Contact Force21/LConn1
  Simscape Bus/LConn20 -- Spatial Contact Force22/LConn1
  Simscape Bus/LConn28 -- Spatial Contact Force16/LConn1
  Simscape Bus/LConn21 -- Spatial Contact Force24/LConn1
  Simscape Bus/LConn25 -- Spatial Contact Force19/LConn1
  Simscape Bus/LConn23 -- Spatial Contact Force23/LConn1
  Simscape Bus/LConn24 -- Spatial Contact Force20/LConn1
  Simscape Bus/LConn16 -- Spatial Contact Force27/LConn1
  Simscape Bus/LConn17 -- Spatial Contact Force26/LConn1
  Simscape Bus/LConn12 -- Spatial Contact Force30/LConn1
  Simscape Bus/LConn10 -- Spatial Contact Force31/LConn1
  Simscape Bus/LConn18 -- Spatial Contact Force25/LConn1
  Simscape Bus/LConn11 -- Spatial Contact Force33/LConn1
  Simscape Bus/LConn15 -- Spatial Contact Force28/LConn1
  Simscape Bus/LConn13 -- Spatial Contact Force32/LConn1
  Simscape Bus/LConn14 -- Spatial Contact Force29/LConn1
  Simscape Bus/LConn6 -- Spatial Contact Force36/LConn1
  Simscape Bus/LConn7 -- Spatial Contact Force35/LConn1
  Simscape Bus/LConn2 -- Spatial Contact Force39/LConn1
  Simscape Bus/LConn8 -- Spatial Contact Force34/LConn1
  Simscape Bus/LConn1 -- Spatial Contact Force42/LConn1
  Simscape Bus/LConn5 -- Spatial Contact Force37/LConn1
  Simscape Bus/LConn3 -- Spatial Contact Force41/LConn1
  Simscape Bus/LConn4 -- Spatial Contact Force38/LConn1
  Spatial Contact Force40/LConn1 -- Simscape Bus/LConn9
  Simscape Bus/LConn19 -- Spatial Contact Force43/LConn1
  Spatial Contact Force47/LConn1 -- Simscape Bus/LConn29
  Simscape Bus/LConn39 -- Spatial Contact Force48/LConn1

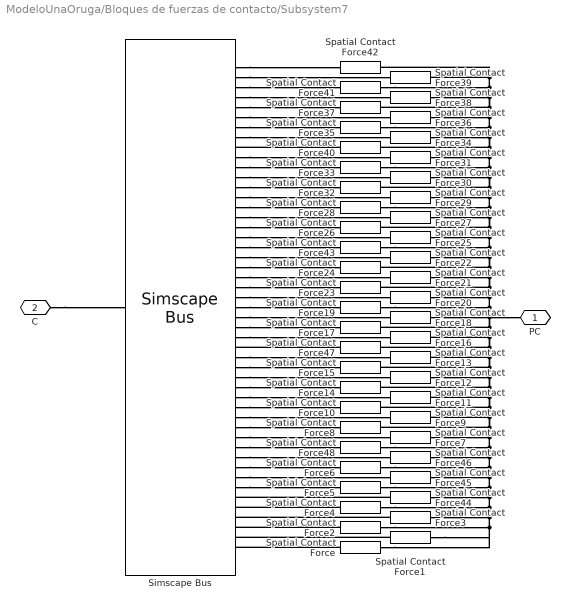
== system ModeloUnaOruga/Bloques de fuerzas de contacto/Subsystem7 ==
  Simscape Bus : SimscapeBus  HierarchyStrings=Connection49;Connection48;Connection47;Connection46;Connection45;Connection44;Connection43;Connection42;Connection41;Connection40;Connection39;Connection38;Connection37;Connection36;Connection35;Connection34;Connection33;Connection32;Connection31;Connection30;Connection29;Connection28;Connection27;Connection26;Connection25;Connection24;Connection23;Connection22;Connection21;Connection20;Connection19;Connection18;Connection17;Connection16;Connection15;Connection14;Connection13;Connection12;Connection11;Connection10;Connection9;Connection8;Connection7;Connection6;Connection5;Connection4;Connection3;Connection2;Connection1
  Spatial Contact Force{,1..48} (49 alike) : sm_lib/Forces and Torques/Spatial Contact Force  SenseContactBaseRotation=off  SenseContactBaseTranslation=off  CoefficientOfDynamicFriction=0.3  CoefficientOfStaticFriction=0.5  NormalDamping=1e3  NormalDampingUnits=N/(m/s)  SenseContactSignal=off  NormalStiffness=1e6  NormalStiffnessUnits=N/m  FrictionalCriticalVelocity=1e-3  FrictionalCriticalVelocityUnits=m/s  ZeroCrossDetectContactStartAndEnd=off  SenseContactFollowerRotation=off  SenseContactFollowerTranslation=off  FrictionType=None  SenseFrictionalForceMagnitude=off  SenseNormalForceMagnitude=off  NormalForceType=SmoothSpringDamper  SenseNormalVelocity=off  SensePenetrationDepth=off  SenseSeparationDistance=off  SenseTangentialVelocity=off  NormalTransitionRegionWidth=1e-4  NormalTransitionRegionWidthUnits=m
  PC : PMIOPort  Side=Right
  C : PMIOPort  Port=2  Side=Left
  connections:
  Spatial Contact Force41/RConn1 -- Spatial Contact Force42/RConn1 -- Spatial Contact Force39/RConn1 -- Spatial Contact Force38/RConn1 -- Spatial Contact Force35/RConn1 -- Spatial Contact Force40/RConn1 -- Spatial Contact Force32/RConn1 -- Spatial Contact Force28/RConn1 -- Spatial Contact Force26/RConn1 -- Spatial Contact Force24/RConn1 -- Spatial Contact Force23/RConn1 -- Spatial Contact Force17/RConn1 -- Spatial Contact Force16/RConn1 -- Spatial Contact Force47/RConn1 -- Spatial Contact Force13/RConn1 -- Spatial Contact Force15/RConn1 -- Spatial Contact Force14/RConn1 -- Spatial Contact Force11/RConn1 -- Spatial Contact Force10/RConn1 -- Spatial Contact Force9/RConn1 -- Spatial Contact Force8/RConn1 -- Spatial Contact Force46/RConn1 -- Spatial Contact Force6/RConn1 -- Spatial Contact Force45/RConn1 -- Spatial Contact Force5/RConn1 -- Spatial Contact Force44/RConn1 -- Spatial Contact Force1/RConn1 -- Spatial Contact Force/RConn1 -- Spatial Contact Force2/RConn1 -- Spatial Contact Force3/RConn1 -- Spatial Contact Force4/RConn1 -- Spatial Contact Force48/RConn1 -- Spatial Contact Force7/RConn1 -- Spatial Contact Force12/RConn1 -- Spatial Contact Force18/RConn1 -- PC/RConn1 -- Spatial Contact Force19/RConn1 -- Spatial Contact Force20/RConn1 -- Spatial Contact Force21/RConn1 -- Spatial Contact Force22/RConn1 -- Spatial Contact Force43/RConn1 -- Spatial Contact Force25/RConn1 -- Spatial Contact Force27/RConn1 -- Spatial Contact Force29/RConn1 -- Spatial Contact Force30/RConn1 -- Spatial Contact Force33/RConn1 -- Spatial Contact Force31/RConn1 -- Spatial Contact Force34/RConn1 -- Spatial Contact Force36/RConn1 -- Spatial Contact Force37/RConn1
  Spatial Contact Force/LConn1 -- Simscape Bus/LConn49
  Spatial Contact Force1/LConn1 -- Simscape Bus/LConn48
  Spatial Contact Force2/LConn1 -- Simscape Bus/LConn47
  Spatial Contact Force3/LConn1 -- Simscape Bus/LConn46
  Spatial Contact Force4/LConn1 -- Simscape Bus/LConn45
  Spatial Contact Force44/LConn1 -- Simscape Bus/LConn44
  Simscape Bus/LConn43 -- Spatial Contact Force5/LConn1
  Simscape Bus/LConn42 -- Spatial Contact Force45/LConn1
  Simscape Bus/LConn41 -- Spatial Contact Force6/LConn1
  Simscape Bus/LConn40 -- Spatial Contact Force46/LConn1
  C/RConn1 -- Simscape Bus/RConn1
  Simscape Bus/LConn36 -- Spatial Contact Force9/LConn1
  Simscape Bus/LConn37 -- Spatial Contact Force8/LConn1
  Simscape Bus/LConn32 -- Spatial Contact Force12/LConn1
  Simscape Bus/LConn30 -- Spatial Contact Force13/LConn1
  Simscape Bus/LConn38 -- Spatial Contact Force7/LConn1
  Simscape Bus/LConn31 -- Spatial Contact Force15/LConn1
  Simscape Bus/LConn35 -- Spatial Contact Force10/LConn1
  Simscape Bus/LConn33 -- Spatial Contact Force14/LConn1
  Simscape Bus/LConn34 -- Spatial Contact Force11/LConn1
  Simscape Bus/LConn26 -- Spatial Contact Force18/LConn1
  Simscape Bus/LConn27 -- Spatial Contact Force17/LConn1
  Simscape Bus/LConn22 -- Spatial Contact Force21/LConn1
  Simscape Bus/LConn20 -- Spatial Contact Force22/LConn1
  Simscape Bus/LConn28 -- Spatial Contact Force16/LConn1
  Simscape Bus/LConn21 -- Spatial Contact Force24/LConn1
  Simscape Bus/LConn25 -- Spatial Contact Force19/LConn1
  Simscape Bus/LConn23 -- Spatial Contact Force23/LConn1
  Simscape Bus/LConn24 -- Spatial Contact Force20/LConn1
  Simscape Bus/LConn16 -- Spatial Contact Force27/LConn1
  Simscape Bus/LConn17 -- Spatial Contact Force26/LConn1
  Simscape Bus/LConn12 -- Spatial Contact Force30/LConn1
  Simscape Bus/LConn10 -- Spatial Contact Force31/LConn1
  Simscape Bus/LConn18 -- Spatial Contact Force25/LConn1
  Simscape Bus/LConn11 -- Spatial Contact Force33/LConn1
  Simscape Bus/LConn15 -- Spatial Contact Force28/LConn1
  Simscape Bus/LConn13 -- Spatial Contact Force32/LConn1
  Simscape Bus/LConn14 -- Spatial Contact Force29/LConn1
  Simscape Bus/LConn6 -- Spatial Contact Force36/LConn1
  Simscape Bus/LConn7 -- Spatial Contact Force35/LConn1
  Simscape Bus/LConn2 -- Spatial Contact Force39/LConn1
  Simscape Bus/LConn8 -- Spatial Contact Force34/LConn1
  Simscape Bus/LConn1 -- Spatial Contact Force42/LConn1
  Simscape Bus/LConn5 -- Spatial Contact Force37/LConn1
  Simscape Bus/LConn3 -- Spatial Contact Force41/LConn1
  Simscape Bus/LConn4 -- Spatial Contact Force38/LConn1
  Spatial Contact Force40/LConn1 -- Simscape Bus/LConn9
  Simscape Bus/LConn19 -- Spatial Contact Force43/LConn1
  Spatial Contact Force47/LConn1 -- Simscape Bus/LConn29
  Simscape Bus/LConn39 -- Spatial Contact Force48/LConn1

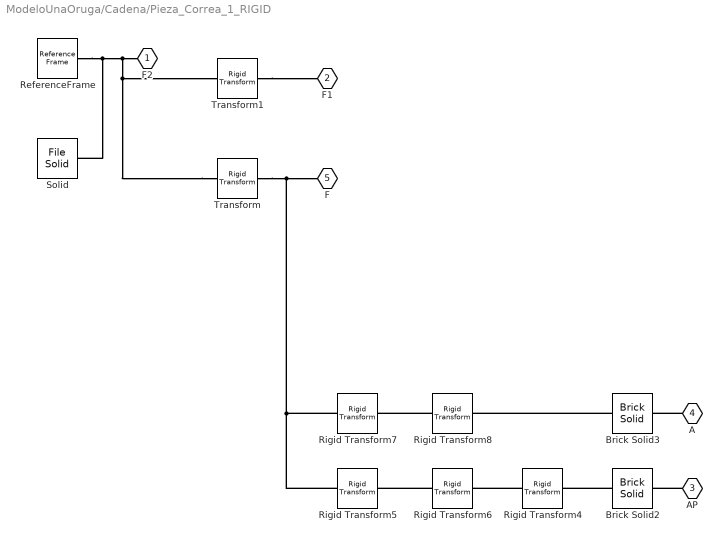
== system ModeloUnaOruga/Cadena/Pieza_Correa_1_RIGID ==
  Brick Solid2 : sm_lib/Body Elements/Brick Solid  GraphicAmbientColor=[0.15 0.15 0.15 1.0]  BasedOnType=Density  BrickDimensions=[4.5 4.5 13]  BrickDimensionsUnits=mm  CenterOfMass=[0 0 0]  CenterOfMassUnits=m  GraphicDiffuseColor=[1.0 0.0 0.0]  Density=1000  DensityUnits=kg/m^3  DoExposeReferenceFrame=on  GraphicEmissiveColor=[0.0 0.0 0.0 1.0]  ExportEntireGeometry=on  SerializedFrames=<Frames/>  MarkerShape=Sphere  MarkerSize=10  GraphicType=None  InertiaType=CalculateFromGeometry  Mass=1  MassUnits=kg  MomentsOfInertia=[1 1 1]  MomentsOfInertiaUnits=kg*m^2  GraphicOpacity=1.0  ProductsOfInertia=[0 0 0]  ProductsOfInertiaUnits=kg*m^2  GraphicShininess=75  GraphicSpecularColor=[0.5 0.5 0.5 1.0]  GraphicVisPropType=SimpleVisualProperties
  Brick Solid3 : sm_lib/Body Elements/Brick Solid  GraphicAmbientColor=[0.15 0.15 0.15 1.0]  BasedOnType=Density  BrickDimensions=[20 5 50]  BrickDimensionsUnits=mm  CenterOfMass=[0 0 0]  CenterOfMassUnits=m  GraphicDiffuseColor=[1.0 0.0 0.0]  Density=1000  DensityUnits=kg/m^3  DoExposeReferenceFrame=on  GraphicEmissiveColor=[0.0 0.0 0.0 1.0]  ExportEntireGeometry=on  SerializedFrames=<Frames/>  MarkerShape=Sphere  MarkerSize=10  GraphicType=None  InertiaType=CalculateFromGeometry  Mass=1  MassUnits=kg  MomentsOfInertia=[1 1 1]  MomentsOfInertiaUnits=kg*m^2  GraphicOpacity=1.0  ProductsOfInertia=[0 0 0]  ProductsOfInertiaUnits=kg*m^2  GraphicShininess=75  GraphicSpecularColor=[0.5 0.5 0.5 1.0]  GraphicVisPropType=SimpleVisualProperties
  ReferenceFrame : sm_lib/Frames and Transforms/Reference Frame
  Rigid Transform4 : sm_lib/Frames and Transforms/Rigid Transform  TranslationMethod=StandardAxis  TranslationStandardOffset=5  TranslationStandardOffsetUnits=mm  TranslationStandardAxis=-Y  TranslationCartesianOffset=[0 0 0]  TranslationCartesianOffsetUnits=m  TranslationROffset=0  TranslationROffsetUnits=m  TranslationZOffset=0  TranslationZOffsetUnits=m  TranslationThetaOffset=0  TranslationThetaOffsetUnits=deg  RotationMethod=None  RotationAngleUnits=deg  RotationStandardAxis=+Z  RotationAngle=0.0  RotationArbitraryAxis=[0 0 1]  FollAlignAxisA=+X  BaseAlignAxisA=+Y  FollAlignAxisB=+Y  BaseAlignAxisB=+Z  RotationSequenceAxes=FollowerAxes  RotationSequence=XYX  RotationSequenceAngles=[0 0 0]  RotationSequenceAnglesUnits=deg  RotationMatrix=[1 0 0; 0 1 0; 0 0 1]  Quaternion=[1 0 0 0]
  Rigid Transform5 : sm_lib/Frames and Transforms/Rigid Transform  TranslationMethod=StandardAxis  TranslationStandardOffset=27  TranslationStandardOffsetUnits=mm  TranslationStandardAxis=-Z  TranslationCartesianOffset=[0 0 0]  TranslationCartesianOffsetUnits=m  TranslationROffset=0  TranslationROffsetUnits=m  TranslationZOffset=0  TranslationZOffsetUnits=m  TranslationThetaOffset=0  TranslationThetaOffsetUnits=deg  RotationMethod=None  RotationAngleUnits=deg  RotationStandardAxis=+Z  RotationAngle=0.0  RotationArbitraryAxis=[0 0 1]  FollAlignAxisA=+X  BaseAlignAxisA=+Y  FollAlignAxisB=+Y  BaseAlignAxisB=+Z  RotationSequenceAxes=FollowerAxes  RotationSequence=XYX  RotationSequenceAngles=[0 0 0]  RotationSequenceAnglesUnits=deg  RotationMatrix=[1 0 0; 0 1 0; 0 0 1]  Quaternion=[1 0 0 0]
  Rigid Transform6 : sm_lib/Frames and Transforms/Rigid Transform  TranslationMethod=StandardAxis  TranslationStandardOffset=10.5  TranslationStandardOffsetUnits=mm  TranslationStandardAxis=-X  TranslationCartesianOffset=[0 0 0]  TranslationCartesianOffsetUnits=m  TranslationROffset=0  TranslationROffsetUnits=m  TranslationZOffset=0  TranslationZOffsetUnits=m  TranslationThetaOffset=0  TranslationThetaOffsetUnits=deg  RotationMethod=None  RotationAngleUnits=deg  RotationStandardAxis=+Z  RotationAngle=0.0  RotationArbitraryAxis=[0 0 1]  FollAlignAxisA=+X  BaseAlignAxisA=+Y  FollAlignAxisB=+Y  BaseAlignAxisB=+Z  RotationSequenceAxes=FollowerAxes  RotationSequence=XYX  RotationSequenceAngles=[0 0 0]  RotationSequenceAnglesUnits=deg  RotationMatrix=[1 0 0; 0 1 0; 0 0 1]  Quaternion=[1 0 0 0]
  Rigid Transform7 : sm_lib/Frames and Transforms/Rigid Transform  TranslationMethod=StandardAxis  TranslationStandardOffset=5  TranslationStandardOffsetUnits=mm  TranslationStandardAxis=+Z  TranslationCartesianOffset=[0 0 0]  TranslationCartesianOffsetUnits=m  TranslationROffset=0  TranslationROffsetUnits=m  TranslationZOffset=0  TranslationZOffsetUnits=m  TranslationThetaOffset=0  TranslationThetaOffsetUnits=deg  RotationMethod=None  RotationAngleUnits=deg  RotationStandardAxis=+Z  RotationAngle=0.0  RotationArbitraryAxis=[0 0 1]  FollAlignAxisA=+X  BaseAlignAxisA=+Y  FollAlignAxisB=+Y  BaseAlignAxisB=+Z  RotationSequenceAxes=FollowerAxes  RotationSequence=XYX  RotationSequenceAngles=[0 0 0]  RotationSequenceAnglesUnits=deg  RotationMatrix=[1 0 0; 0 1 0; 0 0 1]  Quaternion=[1 0 0 0]
  Rigid Transform8 : sm_lib/Frames and Transforms/Rigid Transform  TranslationMethod=StandardAxis  TranslationStandardOffset=12  TranslationStandardOffsetUnits=mm  TranslationStandardAxis=-X  TranslationCartesianOffset=[0 0 0]  TranslationCartesianOffsetUnits=m  TranslationROffset=0  TranslationROffsetUnits=m  TranslationZOffset=0  TranslationZOffsetUnits=m  TranslationThetaOffset=0  TranslationThetaOffsetUnits=deg  RotationMethod=None  RotationAngleUnits=deg  RotationStandardAxis=+Z  RotationAngle=0.0  RotationArbitraryAxis=[0 0 1]  FollAlignAxisA=+X  BaseAlignAxisA=+Y  FollAlignAxisB=+Y  BaseAlignAxisB=+Z  RotationSequenceAxes=FollowerAxes  RotationSequence=XYX  RotationSequenceAngles=[0 0 0]  RotationSequenceAnglesUnits=deg  RotationMatrix=[1 0 0; 0 1 0; 0 0 1]  Quaternion=[1 0 0 0]
  Solid : sm_lib/Body Elements/File Solid  ExtGeomFileName=Pieza Correa_Default_sldprt.STEP  UnitType=FromFile  ExtGeomFileUnits=m  StepReaderType=HEX  ExportConvexHullGeometry=off  InertiaType=Custom  Mass=smiData.Solid(1).mass  MassUnits=kg  CenterOfMass=smiData.Solid(1).CoM  CenterOfMassUnits=mm  MomentsOfInertia=smiData.Solid(1).MoI  MomentsOfInertiaUnits=kg*mm^2  ProductsOfInertia=smiData.Solid(1).PoI  ProductsOfInertiaUnits=kg*mm^2  BasedOnType=DensityFromFile  Density=1000  DensityUnits=kg/m^3  DoExposeReferenceFrame=on  SerializedFrames=<Frames/>  GraphicType=FromGeometry  MarkerShape=Sphere  MarkerSize=10  GraphicVisPropType=SimpleVisualProperties  GraphicDiffuseColor=smiData.Solid(1).color  GraphicSpecularColor=[0.5 0.5 0.5 1.0]  GraphicAmbientColor=[0.15 0.15 0.15 1.0]  GraphicEmissiveColor=[0.0 0.0 0.0 1.0]  GraphicShininess=75  GraphicOpacity=smiData.Solid(1).opacity
  Transform : sm_lib/Frames and Transforms/Rigid Transform  TranslationMethod=Cartesian  TranslationStandardOffset=0  TranslationStandardOffsetUnits=m  TranslationStandardAxis=+Z  TranslationCartesianOffset=smiData.RigidTransform(9).translation  TranslationCartesianOffsetUnits=mm  TranslationROffset=0  TranslationROffsetUnits=m  TranslationZOffset=0  TranslationZOffsetUnits=m  TranslationThetaOffset=0  TranslationThetaOffsetUnits=deg  RotationMethod=ArbitraryAxis  RotationAngleUnits=rad  RotationStandardAxis=+Z  RotationAngle=smiData.RigidTransform(9).angle  RotationArbitraryAxis=smiData.RigidTransform(9).axis  FollAlignAxisA=+X  BaseAlignAxisA=+Y  FollAlignAxisB=+Y  BaseAlignAxisB=+Z  RotationSequenceAxes=FollowerAxes  RotationSequence=XYX  RotationSequenceAngles=[0 0 0]  RotationSequenceAnglesUnits=deg  RotationMatrix=[1 0 0; 0 1 0; 0 0 1]  Quaternion=[1 0 0 0]
  Transform1 : sm_lib/Frames and Transforms/Rigid Transform  TranslationMethod=Cartesian  TranslationStandardOffset=0  TranslationStandardOffsetUnits=m  TranslationStandardAxis=+Z  TranslationCartesianOffset=smiData.RigidTransform(11).translation  TranslationCartesianOffsetUnits=mm  TranslationROffset=0  TranslationROffsetUnits=m  TranslationZOffset=0  TranslationZOffsetUnits=m  TranslationThetaOffset=0  TranslationThetaOffsetUnits=deg  RotationMethod=ArbitraryAxis  RotationAngleUnits=rad  RotationStandardAxis=+Z  RotationAngle=smiData.RigidTransform(11).angle  RotationArbitraryAxis=smiData.RigidTransform(11).axis  FollAlignAxisA=+X  BaseAlignAxisA=+Y  FollAlignAxisB=+Y  BaseAlignAxisB=+Z  RotationSequenceAxes=FollowerAxes  RotationSequence=XYX  RotationSequenceAngles=[0 0 0]  RotationSequenceAnglesUnits=deg  RotationMatrix=[1 0 0; 0 1 0; 0 0 1]  Quaternion=[1 0 0 0]
  F2 : PMIOPort  Side=Left
  F1 : PMIOPort  Port=2  Side=Left
  AP : PMIOPort  Port=3  Side=Right
  A : PMIOPort  Port=4  Side=Right
  F : PMIOPort  Port=5  Side=Right
  connections:
  Transform/LConn1 -- Transform1/LConn1 -- ReferenceFrame/RConn1 -- Solid/RConn1 -- F2/RConn1
  Rigid Transform5/RConn1 -- Rigid Transform7/RConn1 -- F/RConn1 -- Transform/RConn1
  Transform1/RConn1 -- F1/RConn1
  A/RConn1 -- Brick Solid3/LConn1
  Rigid Transform8/RConn1 -- Rigid Transform7/LConn1
  Rigid Transform4/RConn1 -- Rigid Transform6/LConn1
  AP/RConn1 -- Brick Solid2/LConn1
  Rigid Transform6/RConn1 -- Rigid Transform5/LConn1
  Brick Solid3/RConn1 -- Rigid Transform8/LConn1
  Brick Solid2/RConn1 -- Rigid Transform4/LConn1
